simulink model "Flexible_Beam"  (R2021a)
settings: Solver=FixedStepAuto  StartTime=0.0  StopTime=10  FixedStep=1e-4  RelTol=1e-3
values from neighbouring files (symbols this model uses):
  A = [0 1 ; -wn1^2 -2*zeta1*wn1]    [Lab6_code.m]
  A1 = [0 1 ; -wn1^2 -2*zeta1*wn1-K*Ka*Kc1*Ks*wn1^2]    [Lab6_code.m]
  A2 = [0 1 ; -wn2^2 -2*zeta2*wn2]    [Lab6_code.m]
  B = [0 ; K*wn1^2]    [Lab6_code.m]
  B1 = [0 ; K*Ka*wn1^2]    [Lab6_code.m]
  B2 = [0 ; wn2^2]    [Lab6_code.m]
  Ka = 10    [Lab6_code.m]
  Kc1 = 0.1256    [Lab6_code.m]
  Kc2 = 0.015    [Lab6_code.m]
  Ks = 100    [Lab6_code.m]
  x0 = 5e-3    (= 0.005)    [Lab6_code.m]
settings Model: Creator=fades  LastModifiedBy=fades

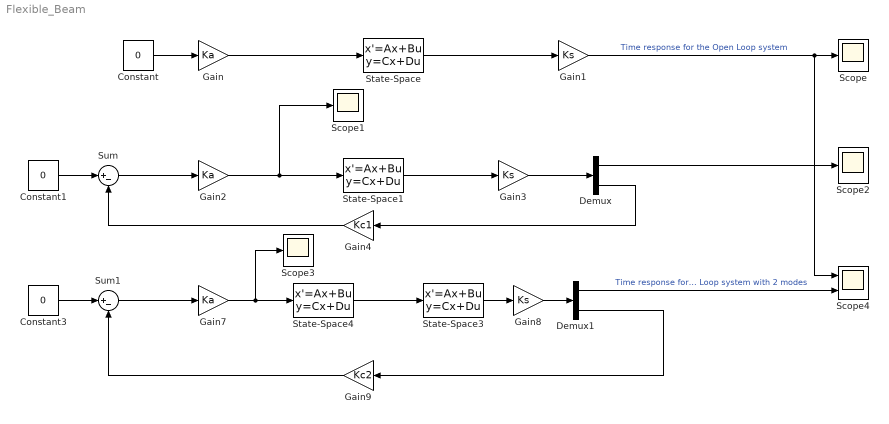
== system Flexible_Beam ==
  Constant : Constant  Value=0
  Constant1 : Constant  Value=0
  Constant3 : Constant  Value=0
  Demux : Demux  Outputs=2
  Demux1 : Demux  Outputs=2
  Gain : Gain  Gain=Ka
  Gain1 : Gain  Gain=Ks
  Gain2 : Gain  Gain=Ka
  Gain3 : Gain  Gain=Ks
  Gain4 : Gain  Gain=Kc1
  Gain7 : Gain  Gain=Ka
  Gain8 : Gain  Gain=Ks
  Gain9 : Gain  Gain=Kc2
  Scope{,1..3} (4 alike) : Scope
  Scope4 : Scope  NumInputPorts=2
  State-Space : StateSpace  A=A  B=B  C=[1 0];  D=0  InitialCondition=[x0 0];
  State-Space1 : StateSpace  A=A1  B=B1  C=[1 0 ; 0 1]  D=zeros(2,1)  InitialCondition=[x0 0];
  State-Space3 : StateSpace  A=A2  B=B2  C=[1 0 ; 0 1]  D=zeros(2,1)  InitialCondition=0
  State-Space4 : StateSpace  A=A  B=B  C=[1 0];  D=0  InitialCondition=[x0 0];
  Sum : Sum  Inputs=|+-
  Sum1 : Sum  Inputs=|+-
  wires:
  Gain/1 -> State-Space/1
  State-Space/1 -> Gain1/1
  Gain1/1 -> Scope4/1, Scope/1  "Time response for the Open Loop system"
  Gain2/1 -> Scope1/1, State-Space1/1
  Sum/1 -> Gain2/1
  State-Space1/1 -> Gain3/1
  Gain3/1 -> Demux/1
  Demux/2 -> Gain4/1
  Gain4/1 -> Sum/2
  Constant/1 -> Gain/1
  Constant1/1 -> Sum/1
  Constant3/1 -> Sum1/1
  Sum1/1 -> Gain7/1
  Gain7/1 -> Scope3/1, State-Space4/1
  State-Space4/1 -> State-Space3/1
  State-Space3/1 -> Gain8/1
  Gain8/1 -> Demux1/1
  Gain9/1 -> Sum1/2
  Demux1/2 -> Gain9/1
  Demux/1 -> Scope2/1
  Demux1/1 -> Scope4/2  "Time response for the Closed Loop system with 2 modes"
